simulink model "FixedImpedance"  (R2024b)
settings: Solver=ode4  StartTime=0.001  StopTime=28  FixedStep=1e-4  RelTol=1e-3
libraries: simulink x4, slpidlib x1
settings Model: PacingRate=2  Creator=edwar  LastModifiedBy=edwar

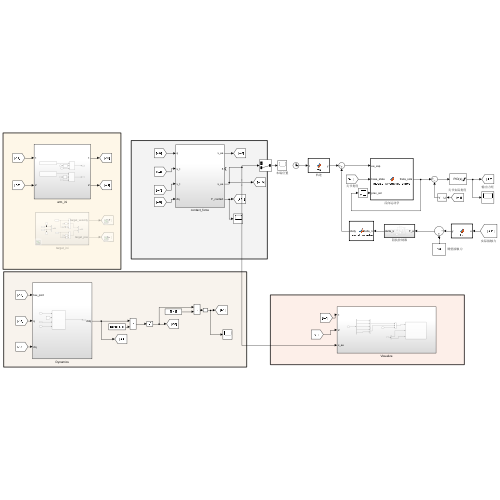
[thumbnail: Simulink's stored preview of the top-level diagram]
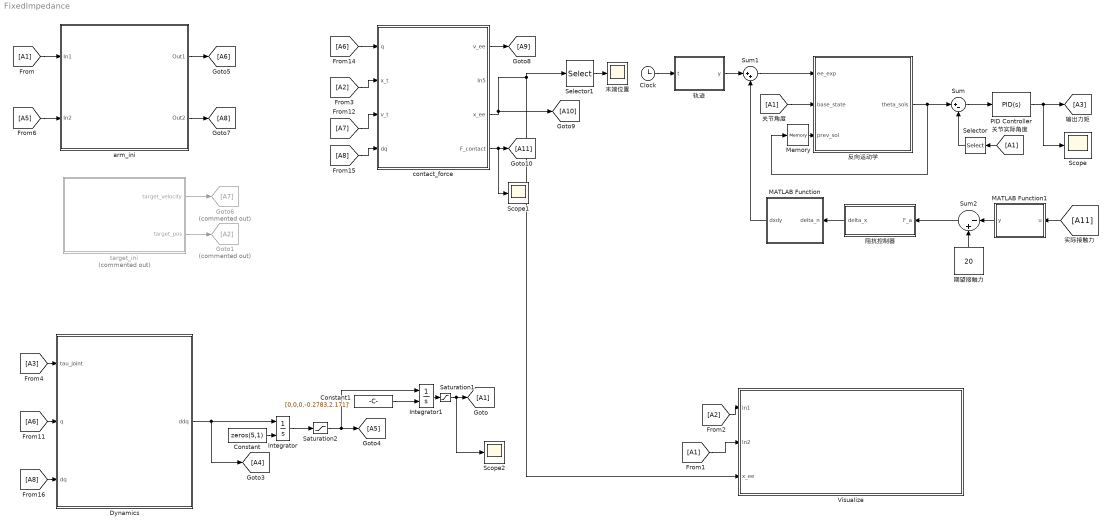
== system FixedImpedance ==
  Clock : Clock
  Constant : Constant  Value=zeros(5,1)
  Constant1 : Constant  Value=[0,0,0,-0.2783,2.171]'
  Dynamics : Subsystem
  Goto1 : Goto  Commented=on  GotoTag=A2
  Goto6 : Goto  Commented=on  GotoTag=A7
  Integrator : Integrator  InitialConditionSource=external  InitialCondition=[0,0,0,0,0]'
  Integrator1 : Integrator  InitialConditionSource=external  InitialCondition=zeros(5,1)
  MATLAB Function : MATLAB Function  TreatAsAtomicUnit=on
  MATLAB Function1 : MATLAB Function  TreatAsAtomicUnit=on
  Memory : Memory  InitialCondition=[0;0]  InheritSampleTime=on
  PID Controller : slpidlib/PID Controller  Controller=PID  Form=Parallel  TimeDomain=Continuous-time  UseExternalTs=off  SampleTime=-1  IntegratorMethod=Forward Euler  FilterMethod=Forward Euler  ControllerParametersSource=internal  P=0.5  I=0  UseKiTs=off  D=0.8  UseExternalDerivativeSource=off  N=100  UseFilter=on  TunerSelectOption=Transfer Function Based (PID Tuner App)  InitialConditionSource=internal  InitialConditionForIntegrator=0  InitialConditionForFilter=0  DifferentiatorICPrevScaledInput=0  ExternalReset=none  TrackingMode=off  Kt=1  LimitOutput=on  SatLimitsSource=internal  UpperSaturationLimit=1.4  LowerSaturationLimit=-1.4  LinearizeAsGain=on  AntiWindupMode=none  Kb=1  LimitIntegrator=off  UpperIntegratorSaturationLimit=inf  LowerIntegratorSaturationLimit=-inf  POutMin=[]  POutMax=[]  IOutMin=[]  IOutMax=[]  DOutMin=[]  DOutMax=[]  NOutMin=[]  NOutMax=[]  SumOutMin=[]  SumOutMax=[]  SaturationOutMin=[]  SaturationOutMax=[]  PParamMin=[]  PParamMax=[]  IParamMin=[]  IParamMax=[]  DParamMin=[]  DParamMax=[]  NParamMin=[]  NParamMax=[]  KbParamMin=[]  KbParamMax=[]  KtParamMin=[]  KtParamMax=[]  KbOutMin=[]  KbOutMax=[]  KtOutMin=[]  KtOutMax=[]  IntegratorOutMin=[]  IntegratorOutMax=[]  FilterOutMin=[]  FilterOutMax=[]  SumI1OutMin=[]  SumI1OutMax=[]  SumI2OutMin=[]  SumI2OutMax=[]  SumI3OutMin=[]  SumI3OutMax=[]  SumI4OutMin=[]  SumI4OutMax=[]  SumDOutMin=[]  SumDOutMax=[]  DifferentiatorOutMin=[]  DifferentiatorOutMax=[]  FilterDiffOutCoefMin=[]  FilterDiffOutCoefMax=[]  ReciprocalOutMin=[]  ReciprocalOutMax=[]  SumDenOutMin=[]  SumDenOutMax=[]  SumNumOutMin=[]  SumNumOutMax=[]  DivideOutMin=[]  DivideOutMax=[]  UdiffTsProdOutMin=[]  UdiffTsProdOutMax=[]  NTsProdOutMin=[]  NTsProdOutMax=[]  UintegralTsProdOutMin=[]  UintegralTsProdOutMax=[]  UngainTsProdOutMin=[]  UngainTsProdOutMax=[]  ClampingZeroOutDataTypeStr=Inherit: Inherit via back propagation  ClampingZeroOutMin=[]  ClampingZeroOutMax=[]  FilterDenConstantOutDataTypeStr=Inherit: Inherit via back propagation  FilterDenConstantOutMin=[]  FilterDenConstantOutMax=[]  PCopyOutDataTypeStr=Inherit: Inherit via back propagation  PCopyOutMin=[]  PCopyOutMax=[]  NCopyOutDataTypeStr=Inherit: Inherit via back propagation  NCopyOutMin=[]  NCopyOutMax=[]  IntegratorContinuousStateAttributes=''  IntegratorStateMustResolveToSignalObject=off  IntegratorRTWStateStorageClass=Auto  FilterContinuousStateAttributes=''  FilterStateMustResolveToSignalObject=off  FilterRTWStateStorageClass=Auto  ParallelPVariant=InternalParameters  IdealPVariant=Disabled  IVariant=InternalParameters  DVariant=InternalParameters  IntegratorVariant=Continuous  SatVariant=Enabled  AWVariant=Passthrough  PCopyVariant=Disabled  TRVariant=Disabled  FdbkBlocksVariant=Forward  IdealPFdbkVariant=Disabled  SatFdbkVariant=Disabled  DerivativeFilterVariant=ContFilter  NVariant=InternalParameters  NCopyVariant=Disabled  FilterICVariant=InternalICsFilter  IntegratorICVariant=InternalICs  ExternalResetVariant=Disabled  TRSumVariant=Passthrough  SumFdbkVariant=Disabled  SumVariant=Sum_PID  TsampFilterVariant=InternalTs  TsampNgainVariant=Passthrough  TsampIntegralVariant=Disabled_SignalSpec  ExternalSaturationOutDataTypeStr=Inherit: Same as second input  DerivativeSourceVariant=ErrorSignal  PreIntVariant=InternalPreInt
  Saturation1 : Saturate  UpperLimit=[1.5,1.5,5*pi,2.5,2.5]'  LowerLimit=[-1.5,-1.5,-5*pi,-2.5,-2.5]'
  Saturation2 : Saturate  UpperLimit=[0.075,0.075,pi/6,4.2,4.2]'  LowerLimit=[-0.075,-0.075,-pi/6,-4.2,-4.2]'
  Scope : Scope
  Scope1 : Scope
  Scope2 : Scope
  Selector : Selector  InputPortWidth=5  IndexOptions=Index vector (dialog)  Indices=[4 5]  OutputSizes=1
  Selector1 : Selector  InputPortWidth=2  IndexOptions=Index vector (dialog)  Indices=[2]  OutputSizes=1
  Sum : Sum  Inputs=|+-
  Sum1 : Sum  Inputs=|++
  Sum2 : Sum  Inputs=|-+
  Visualize : Subsystem
  arm_ini : Subsystem
  contact_force : Subsystem
      settings: PortSchema="{\"entries\":[{\"content\":{\"sides\":[{\"content\":{\"connectorIds\":[\"In1\",\"In2\",\"In3\",\"In4\"]},\"type\":\"ConnectorPlacement.EquallySpacedRectSide\",\"uuid\":\"4288fde3-8199-4324-a6f9-6cd5d2cca29d\"},{\"content\":{\"connectorIds\":[\"Out1\",\"In5\",\"Out2\",\"Out3\"],\"side\":\"RIGHT\"},\"type\":\"ConnectorPlacement.EquallySpacedRectSide\",\"uuid\":\"5c78b4d8-bb77-466a-a925-fe5a2b505b9a\"},{\"content\":{\"side\":\"TOP\"},\"type\":\"ConnectorPlacement.EquallySpacedRectSide\",\"uuid\":\"fef07971-ef14-435e-90c8-30ad3be9ea68\"}]},\"type\":\"ConnectorPlacement.EquallySpacedConnector\",\"uuid\":\"c2bdddc2-d220-4e31-8d95-6807f4723718\"}],\"packageUris\":[\"http://schema.mathworks.com/mf0/Connector/R2020b\"],\"version\":\"1.0\"}"
  target_ini : Subsystem  Commented=on
  反向运动学 : MATLAB Function  TreatAsAtomicUnit=on
  期望接触力 : Constant  Value=20
  末端位置 : Scope
  轨迹 : MATLAB Function  TreatAsAtomicUnit=on
  阻抗控制器 : Subsystem  TreatAsAtomicUnit=on
  wires:
  Saturation2/1 -> Integrator1/1, [A5]
  Saturation1/1 -> Scope2/1, [A1]
  Constant1/1 -> Integrator1/2
  Constant/1 -> Integrator/2
  Integrator1/1 -> Saturation1/1
  Integrator/1 -> Saturation2/1
  Dynamics/1(ddq) -> [A4], Integrator/1
  [A1] -> arm_ini/1(In1)
  [A1] -> Visualize/2(In2)
  [A2] -> Visualize/1(In1)
  [A3] -> Dynamics/1(tau_joint)
  [A5] -> arm_ini/2(In2)
  [A2] -> contact_force/2(x_t)
  target_ini/1(target_velocity) -> Goto6/1
  [A7] -> contact_force/3(v_t)
  target_ini/2(target_pos) -> Goto1/1
  arm_ini/1(Out1) -> [A6]
  [A6] -> Dynamics/2(q)
  [A6] -> contact_force/1(q)
  arm_ini/2(Out2) -> [A8]
  [A8] -> contact_force/4(dq)
  [A8] -> Dynamics/3(dq)
  contact_force/1(v_ee) -> [A9]
  contact_force/2(x_ee) -> Selector1/1, Visualize/3(x_ee), [A10]
  contact_force/3(F_contact) -> Scope1/1, [A11]
  PID Controller/1 -> [A3], Scope/1
  Sum/1 -> PID Controller/1
  [A1] -> Selector/1
  [A1] -> 反向运动学/2(base_state)
  Selector/1 -> Sum/2
  反向运动学/1(theta_sols) -> Memory/1, Sum/1
  阻抗控制器/1(delta_x) -> MATLAB Function/1(delta_n)
  Sum1/1 -> 反向运动学/1(ee_exp)
  [A11] -> MATLAB Function1/1(u)
  期望接触力/1 -> Sum2/2
  Sum2/1 -> 阻抗控制器/1(F_a)
  轨迹/1(y) -> Sum1/1
  Clock/1 -> 轨迹/1(t)
  Memory/1 -> 反向运动学/3(prev_sol)
  MATLAB Function1/1(y) -> Sum2/1
  MATLAB Function/1(dxdy) -> Sum1/2
  Selector1/1 -> 末端位置/1

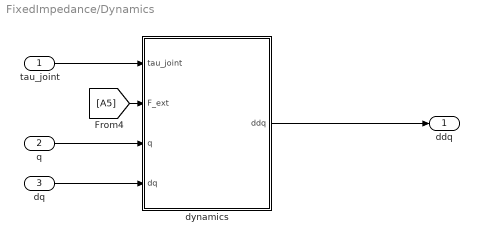
== system FixedImpedance/Dynamics ==
  tau_joint : Inport
  q : Inport  Port=2
  dq : Inport  Port=3
  dynamics : MATLAB Function  TreatAsAtomicUnit=on
  ddq : Outport
  wires:
  tau_joint/1 -> dynamics/1(tau_joint)
  [A5] -> dynamics/2(F_ext)
  dq/1 -> dynamics/4(dq)
  dynamics/1(ddq) -> ddq/1
  q/1 -> dynamics/3(q)

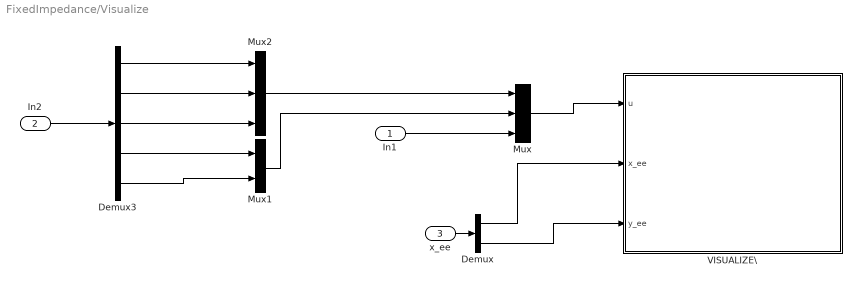
== system FixedImpedance/Visualize ==
  In1 : Inport
  In2 : Inport  Port=2
  x_ee : Inport  Port=3
  Demux : Demux  Outputs=2
  Demux3 : Demux  Outputs=5
  Mux : Mux  Inputs=3
  Mux1 : Mux  Inputs=2
  Mux2 : Mux  Inputs=3
  VISUALIZE\ : MATLAB Function  TreatAsAtomicUnit=on
  wires:
  Demux3/4 -> Mux1/1
  Mux/1 -> VISUALIZE\/1(u)
  Demux3/3 -> Mux2/3
  Mux2/1 -> Mux/1
  Demux3/2 -> Mux2/2
  Mux1/1 -> Mux/2
  Demux3/5 -> Mux1/2
  Demux3/1 -> Mux2/1
  In1/1 -> Mux/3
  In2/1 -> Demux3/1
  x_ee/1 -> Demux/1
  Demux/2 -> VISUALIZE\/3(y_ee)
  Demux/1 -> VISUALIZE\/2(x_ee)

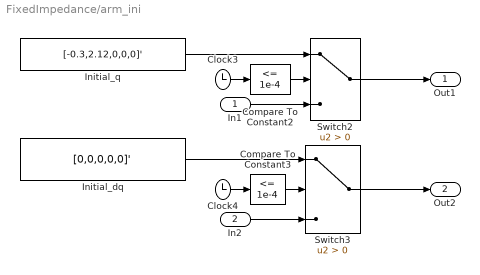
== system FixedImpedance/arm_ini ==
  In1 : Inport
  In2 : Inport  Port=2
  Clock3 : Clock
  Clock4 : Clock
  Compare To Constant2 : simulink/Logic and Bit Operations/Compare To Constant  relop=<=  const=1e-4  OutDataTypeStr=boolean
  Compare To Constant3 : simulink/Logic and Bit Operations/Compare To Constant  relop=<=  const=1e-4  OutDataTypeStr=boolean
  Initial_dq : Constant  Value=[0,0,0,0,0]'
  Initial_q : Constant  Value=[-0.3,2.12,0,0,0]'
  Switch2 : Switch  Criteria=u2 > Threshold  SaturateOnIntegerOverflow=off  InputSameDT=off
  Switch3 : Switch  Criteria=u2 > Threshold  SaturateOnIntegerOverflow=off  InputSameDT=off
  Out1 : Outport
  Out2 : Outport  Port=2
  wires:
  In1/1 -> Switch2/3
  Compare To Constant3/1 -> Switch3/2
  Switch3/1 -> Out2/1
  Initial_dq/1 -> Switch3/1
  Clock3/1 -> Compare To Constant2/1
  In2/1 -> Switch3/3
  Clock4/1 -> Compare To Constant3/1
  Initial_q/1 -> Switch2/1
  Compare To Constant2/1 -> Switch2/2
  Switch2/1 -> Out1/1

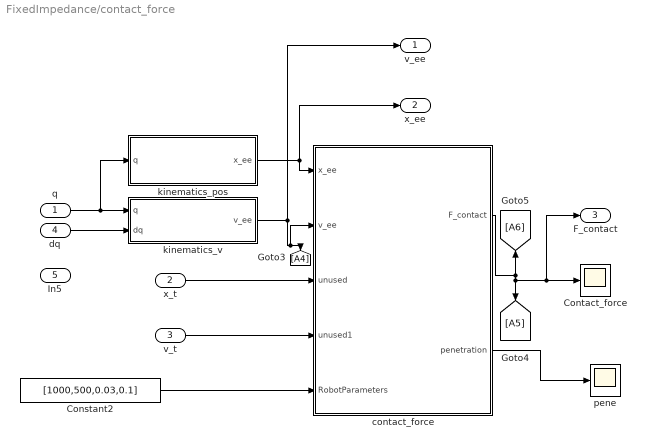
== system FixedImpedance/contact_force ==
  q : Inport
  x_t : Inport  Port=2
  v_t : Inport  Port=3
  dq : Inport  Port=4
  In5 : Inport  Port=5
  Constant2 : Constant  Value=[1000,500,0.03,0.1]
  Contact_force : Scope
  contact_force : MATLAB Function  TreatAsAtomicUnit=on  SystemSampleTime=0.01
  kinematics_pos : MATLAB Function  TreatAsAtomicUnit=on
  kinematics_v : MATLAB Function  TreatAsAtomicUnit=on
  pene : Scope
  v_ee : Outport
  x_ee : Outport  Port=2
  F_contact : Outport  Port=3
  wires:
  kinematics_v/1(v_ee) -> v_ee/1, contact_force/2(v_ee), [A4]
  contact_force/1(F_contact) -> [A5], Contact_force/1, F_contact/1, [A6]
  kinematics_pos/1(x_ee) -> x_ee/1, contact_force/1(x_ee)
  x_t/1 -> contact_force/3(unused)
  Constant2/1 -> contact_force/5(RobotParameters)
  q/1 -> kinematics_pos/1(q), kinematics_v/1(q)
  v_t/1 -> contact_force/4(unused1)
  dq/1 -> kinematics_v/2(dq)
  contact_force/2(penetration) -> pene/1

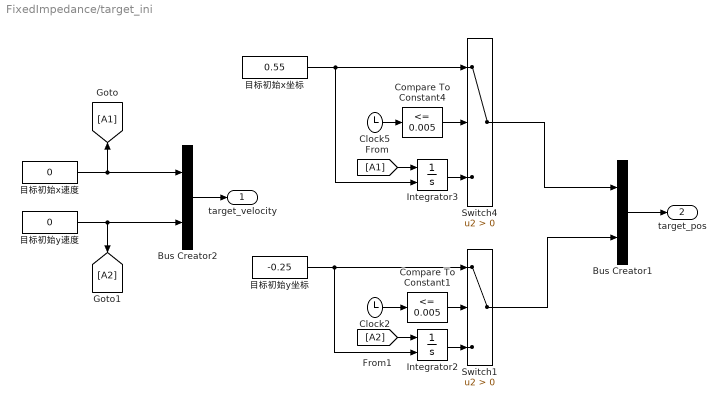
== system FixedImpedance/target_ini ==
  Bus Creator1 : BusCreator  Inputs=2
  Bus Creator2 : BusCreator  Inputs=2
  Clock2 : Clock
  Clock5 : Clock
  Compare To Constant1 : simulink/Logic and Bit Operations/Compare To Constant  relop=<=  const=0.005  OutDataTypeStr=boolean
  Compare To Constant4 : simulink/Logic and Bit Operations/Compare To Constant  relop=<=  const=0.005  OutDataTypeStr=boolean
  Integrator2 : Integrator  InitialConditionSource=external
  Integrator3 : Integrator  InitialConditionSource=external
  Switch1 : Switch  Criteria=u2 > Threshold  SaturateOnIntegerOverflow=off  InputSameDT=off
  Switch4 : Switch  Criteria=u2 > Threshold  SaturateOnIntegerOverflow=off  InputSameDT=off
  目标初始x坐标 : Constant  Value=0.55
  目标初始x速度 : Constant  Value=0
  目标初始y坐标 : Constant  Value=-0.25
  目标初始y速度 : Constant  Value=0
  target_velocity : Outport
  target_pos : Outport  Port=2
  wires:
  Compare To Constant4/1 -> Switch4/2
  Integrator2/1 -> Switch1/3
  Integrator3/1 -> Switch4/3
  目标初始x速度/1 -> [A1], Bus Creator2/1
  目标初始x坐标/1 -> Switch4/1, Integrator3/2
  目标初始y坐标/1 -> Switch1/1, Integrator2/2
  目标初始y速度/1 -> [A2], Bus Creator2/2
  Compare To Constant1/1 -> Switch1/2
  Switch4/1 -> Bus Creator1/1
  Clock5/1 -> Compare To Constant4/1
  Clock2/1 -> Compare To Constant1/1
  Switch1/1 -> Bus Creator1/2
  Bus Creator2/1 -> target_velocity/1
  Bus Creator1/1 -> target_pos/1
  [A1] -> Integrator3/1
  [A2] -> Integrator2/1

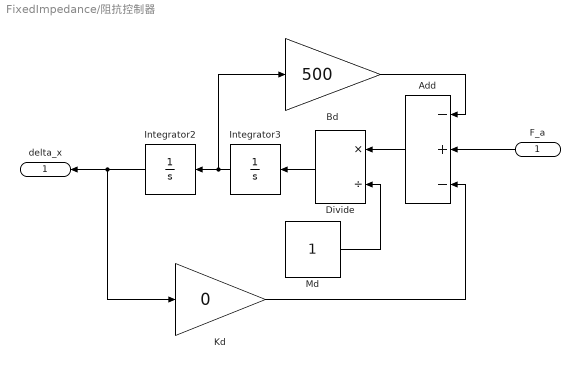
== system FixedImpedance/阻抗控制器 ==
  F_a : Inport
  Add : Sum  Inputs=-+-
  Bd : Gain  Gain=500
  Divide : Product  Inputs=*/
  Integrator2 : Integrator
  Integrator3 : Integrator
  Kd : Gain  Gain=0
  Md : Constant
  delta_x : Outport
  wires:
  Md/1 -> Divide/2
  Bd/1 -> Add/1
  Integrator3/1 -> Integrator2/1, Bd/1
  Kd/1 -> Add/3
  Add/1 -> Divide/1
  F_a/1 -> Add/2
  Integrator2/1 -> delta_x/1, Kd/1
  Divide/1 -> Integrator3/1

== matlab function FixedImpedance/Dynamics/dynamics ==
  data: tau_joint input; F_ext input size=[2,1]; q input size=[5,1]; ddq output size=[5,1]; dq input size=[5,1]
function ddq  = robot_dynamics(tau_joint, F_ext, q, dq)
    % 平面二连杆机器人动力学模型
    % 输入: tau_joint (2x1), F_ext (2x1?), q (5x1), dq (5x1?)
    % 输出: ddq (5x1)


    % 构建力矩向量（5维，前三个分量为0，假设前3是基座自由度不受控）
    tau_control = zeros(5,1);
    tau_control(4:5) = tau_joint(:);  % 关节控制力矩

    J = jacobian_matrix(q);

    % 接触力映射到关节空间
    if ~isempty(F_ext)
        tau_contact = -J' * F_ext(:);
    else
        tau_contact = zeros(5,1);
    end

    tau_total = tau_control + tau_contact;
    damping_coeff = 0.05;  % 0.02 ~ 0.1
    tau_damping = -damping_coeff * dq;  % 5x1，对所有自由度加线性阻尼
    tau_total = tau_total + tau_damping;
    [D, C] = dynamics_model(q, dq); 
    det_D = det(D);
    cond_D = cond(D);
    % 加速度
    ddq = D \ (tau_total - C);
end

== matlab function FixedImpedance/contact_force/kinematics_pos ==
  data: x_ee output; q input
function x_ee  = forward_kinematics(q)
    x_ee = zeros(1,2);
    % q = [x_b; y_b; theta_b; theta1; theta2]
    x_b = q(1); y_b = q(2); theta_b = q(3);
    theta1 = q(4); theta2 = q(5);
    b_b = 0.151;
    L1 = 0.225; L2 = 0.276;  % 连杆长度
    
    % 相对基座的末端位置
    x_rel = b_b + L1*cos(theta1) + L2*cos(theta1+theta2);
    y_rel = L1*sin(theta1) + L2*sin(theta1+theta2);
    
    % 转换到世界坐标系
    R = [cos(theta_b) -sin(theta_b); sin(theta_b) cos(theta_b)];
    pos_world = R * [x_rel; y_rel] + [x_b; y_b];
    
    x_ee(1) = pos_world(1);
    x_ee(2) = pos_world(2);
end

== matlab function FixedImpedance/contact_force/contact_force ==
  data: x_ee input; F_contact output double size=[2,1]; v_ee input; unused input; unused1 input; RobotParameters input; penetration output
function [F_contact,penetration] = contact_force(x_ee, v_ee, ~, ~, RobotParameters)
    % 预分配接触力
    F_contact = zeros(2,1);   
    x_ee = x_ee(:);
    v_ee = v_ee(:);
    
    % 提取参数
    K    = RobotParameters(1);
    B    = RobotParameters(2);
    R_ee = RobotParameters(3); % 末端工具半径
    
    %% 正弦曲面参数 (固定墙体在上方，高度带有 0.2 偏移)

    y = x_ee(2);
    
    %% 1. 计算当前 X 位置对应的曲面 Y 高度
    % 纯 Y 方向模型不需要计算导数 dydx 了
    y_surface = 0.2;
    
    %% 2. 计算纯 Y 方向的穿透深度
    % 机械臂在下方，最上沿的坐标是 y + R_ee
    % 当最上沿超过曲面高度时，发生接触
    penetration = (y + R_ee) - y_surface;
    
    if penetration > 0
        %% 3. 计算沿 Y 方向挤压墙体的速度
        % v_ee(2) 是末端在世界坐标系 Y 方向的速度
        % 因为墙在上方，向上运动（vy > 0）代表正在挤入墙体
        v_in = v_ee(2); 
        
        %% 4. 计算接触力的大小
        F_spring = K * penetration;
        F_damp   = B * max(v_in, 0); % 只有向上挤压墙体时才产生阻尼力
        
        %% 5. 输出接触力向量（方向绝对沿世界坐标 Y 轴向下）
        % 墙体在上方，给机械臂的弹力与阻尼力必然是垂直向下的
        F_contact(1) = 0;                  % X 方向不受力
        F_contact(2) = -(F_spring + F_damp); % Y 方向受力向下
    end
end

== matlab function FixedImpedance/contact_force/kinematics_v ==
  data: q input; v_ee output; dq input
function v_ee = forward_kinematics_v(q,dq)
J = jacobian_matrix(q);
% 计算末端速度
v_ee = (J * dq)';
end

== matlab function FixedImpedance/Visualize/VISUALIZE\ ==
  settings: updateMethod=DISCRETE
  data: u input; x_ee input; y_ee input
function visualize_arm(u,x_ee,y_ee)

% ================================================
% 平面二连杆自由基座机械臂 + 水平墙面 可视化（Simulink专用）
% 输入 u = [x_b, y_b, theta_b, q1, q2, x_ee, y_ee]
%       前5个：用于绘制机械臂本体
%       后2个：直接传入的末端执行器位置，用于绘制轨迹
% ================================================

% ================== 参数（直接使用您提供的值） ==================
b_b   = 0.151;   % 基座质心到关节1距离 (m)
l1    = 0.225;   % 连杆1长度 (m)
l2    = 0.276;   % 连杆2长度 (m)
R_ee  = 0.03;    % 末端执行器半径 (m)

% ================== 持久化图形对象（只创建一次） ==================
persistent h_fig h_base h_link1 h_link2 h_ee h_surface ...
           ee_offset_x ee_offset_y base_vertices
persistent call_counter visualize_every
persistent h_traj traj_x traj_y max_traj_points traj_idx  % 轨迹相关

if isempty(call_counter)
    call_counter = 0;
    visualize_every = 50;
end

call_counter = call_counter + 1;
if mod(call_counter, visualize_every) ~= 0
    return;
end

if isempty(h_fig)
    h_fig = figure();
    ax = gca;
    hold(ax, 'on');
    grid(ax, 'on');
    axis(ax, 'equal');
    xlim(ax, [-0.5 1]);
    ylim(ax, [-0.5 1]);
    xlabel(ax, 'X (m)');
    ylabel(ax, 'Y (m)');
    
    % 初始化基座线段
    base_size = 0.28;           
    half = base_size / 2;
    base_vertices = [ ...
        -half, -half;
         half, -half;
         half,  half;
        -half,  half;
        -half, -half];
    
    % 创建基座
    h_base = patch(ax, ...
        'XData', base_vertices(:,1), 'YData', base_vertices(:,2), ...
        'FaceColor', 'k', ...     
        'EdgeColor', [0.5 0.5 0.5], ...            
        'LineWidth', 2.5, ...
        'FaceAlpha', 0.85);
        
    h_link1 = line(ax, [0 0], [0 0], 'Color', [0.5 0.5 0.5], 'LineWidth', 4, 'DisplayName', 'L1');
    h_link2 = line(ax, [0 0], [0 0], 'Color', [0.5 0.5 0.5], 'LineWidth', 4, 'DisplayName', 'L2');
    
    % 末端执行器圆圈
    theta_c = linspace(0, 2*pi, 50);
    ee_offset_x = R_ee * cos(theta_c);
    ee_offset_y = R_ee * sin(theta_c);
    h_ee = line(ax, ee_offset_x, ee_offset_y, ...
                'Color', 'b', 'LineWidth', 1.5);
                     
    x_surface = linspace(-0.5, 1, 500);
    y_surface = 0.2;
    h_surface = line(ax, x_surface, y_surface, ...
                     'Color', 'k', ...         % 'r' 改为 'k' (黑色)
                     'LineStyle', '--', ...    % 新增：设置为虚线
                     'LineWidth', 1.5);
    
    % 【新增】初始化轨迹线
    h_traj = line(ax, nan, nan, ...
                  'Color', [0 0 1], ...      % 深绿色
                  'LineWidth', 1.5, ...
                  'LineStyle', '--');
    
    % 【新增】初始化轨迹存储
    max_traj_points = 10000;
    traj_x = nan(max_traj_points, 1);
    traj_y = nan(max_traj_points, 1);
    traj_idx = 1;
    
end

% ================== 提取输入 ==================
xb     = u(1);
yb     = u(2);
thetab = u(3);
q1     = u(4);
q2     = u(5);


% ================== 正运动学（用于绘制连杆，不含末端） ==================
x_j1 = xb + b_b * cos(thetab);
y_j1 = yb + b_b * sin(thetab);
x_j2 = x_j1 + l1 * cos(thetab + q1);
y_j2 = y_j1 + l1 * sin(thetab + q1);
% 注意：这里不再计算 x_ee, y_ee，而是直接使用传入的

% ================== 更新轨迹（使用传入的末端位置） ==================
traj_x(traj_idx) = x_ee;
traj_y(traj_idx) = y_ee;

traj_idx = traj_idx + 1;
if traj_idx > max_traj_points
    traj_idx = 1;
end

% 获取有效轨迹数据
if traj_idx > 1
    valid_x = traj_x(1:traj_idx-1);
    valid_y = traj_y(1:traj_idx-1);
else
    valid_x = traj_x;
    valid_y = traj_y;
end
set(h_traj, 'XData', valid_x, 'YData', valid_y);

% ================== 更新图形 ==================
R = [cos(thetab), -sin(thetab); 
     sin(thetab),  cos(thetab)];
 
rotated = (R * base_vertices')';          
abs_x = xb + rotated(:,1);
abs_y = yb + rotated(:,2);

set(h_base, 'XData', abs_x, 'YData', abs_y);
set(h_link1, 'XData', [x_j1, x_j2], 'YData', [y_j1, y_j2]);
set(h_link2, 'XData', [x_j2, x_ee], 'YData', [y_j2, y_ee]);  % 使用传入的末端位置
set(h_ee,    'XData', x_ee + ee_offset_x, 'YData', y_ee + ee_offset_y);  % 使用传入的末端位置

drawnow limitrate;

end

== matlab function FixedImpedance/反向运动学 ==
  data: ee_exp input; theta_sols output; base_state input; prev_sol input
function theta_sols = inverse_kinematics_stable(ee_exp, base_state, prev_sol)
    %#codegen
    b_b = 0.151; L1 = 0.225; L2 = 0.276;
    
    x_t = ee_exp(1); y_t = ee_exp(2);
    x_b = base_state(1); y_b = base_state(2); theta_b = base_state(3);
    
    % 当前关节角（带保护）
    if length(base_state) >= 5
        q_current = [base_state(4); base_state(5)];
    else
        q_current = [0; 0];
    end
    
    % 使用上一次成功解作为参考，确保是列向量
    if nargin < 3 || isempty(prev_sol)
        ref = q_current(:);  % 确保是列向量
    else
        ref = prev_sol(:);   % 确保是列向量
    end
   
    
    % 坐标变换
    dx = x_t - x_b; dy = y_t - y_b;
    x_prime = cos(theta_b)*dx + sin(theta_b)*dy - b_b;
    y_prime = -sin(theta_b)*dx + cos(theta_b)*dy;
    
    r_sq = x_prime^2 + y_prime^2;
    r = sqrt(r_sq);
    
    % 可达性检查
    if r > (L1 + L2) || r < abs(L1 - L2) || r < 1e-6
        theta_sols = ref(:);  % 确保输出是列向量
        return;
    end
    
    cos_theta2 = (r_sq - L1^2 - L2^2) / (2 * L1 * L2);
    cos_theta2 = max(-1.0, min(1.0, cos_theta2));
    
    sin_theta2 = sqrt(1 - cos_theta2^2);   % 正值
    
    angle_base = atan2(y_prime, x_prime);
    
    % 两组解（确保都是列向量）
    theta2_a = atan2( sin_theta2, cos_theta2);
    theta2_b = atan2(-sin_theta2, cos_theta2);
    
    theta1_a = angle_base - atan2(L2*sin_theta2, L1 + L2*cos_theta2);
    theta1_b = angle_base - atan2(-L2*sin_theta2, L1 + L2*cos_theta2);
    
    sol_a = [theta1_a; theta2_a];
    sol_b = [theta1_b; theta2_b];
    
    % ================== 关键改进：连续性处理 ==================
    % 1. 先把两组解都缠绕到最接近参考解
    sol_a = ref + wrapToPi(sol_a - ref);
    sol_b = ref + wrapToPi(sol_b - ref);
    
    % 2. 计算代价（距离 + 配置切换惩罚）
    % 现在ref(1)和ref(2)都可以安全访问
    cost_a = sum((sol_a - ref).^2) + 0.5 * abs(sol_a(2) - ref(2));
    cost_b = sum((sol_b - ref).^2) + 0.5 * abs(sol_b(2) - ref(2));  
    % 3. 优先选择最接近的
    if cost_a <= cost_b
        theta_sols = sol_a;
    else
        theta_sols = sol_b;
    end
    
    % 最终再对当前状态做一次小调整（防止累计漂移）
    theta_sols = ref + wrapToPi(theta_sols - ref);
    theta_sols = theta_sols(:);  % 确保输出是列向量
end

== matlab function FixedImpedance/MATLAB Function ==
  data: delta_n input; dxdy output
function dxdy = sinusoidal_impedance(delta_n)
    dxdy = zeros(2, 1);
%#codegen

    % X 方向不作任何阻抗修正，防止前进方向死锁
    dxdy(1) = 0; 
    
    % Y 方向直接赋修正量
    % 注：如果你的 delta_n 物理意义是指向“上方”为正，而你想让它往下压，这里可以加负号（-delta_n）
    dxdy(2) = delta_n; 
    
end
% % 正弦曲线接触面的阻抗修正
%     %
%     % 输入:
%     %   delta_n - 法向修正量（标量）
%     %   x_t, y_t - 实际末端位置（世界坐标）
%     %   x_b, y_b, theta_b - 基座状态
%     %   b_b - 基座偏移
%     %   A - 正弦曲线幅值
%     %   omega - 正弦曲线频率
%     %   phi - 正弦曲线相位
%     %
%     % 输出:
%     %   dx, dy - XY方向修正量（世界坐标）
% 
% 
% function dxdy = sinusoidal_impedance(delta_n, ee_target,base_state)
%     dxdy=zeros(2,1);
% %#codegen
%     % 简化版：直接计算当前x位置的法向量
%     x_b = base_state(1);
%     y_b = base_state(2);
%     theta_b = base_state(3);
%     b_b = 0.151;
%     omega = 2*pi/0.3;
%     A = 0.05;
%     phi = 0;
%     x_t = ee_target(1);
%     y_t = ee_target(2);
%     % 转换到基座坐标系
%     dx_world = x_t - x_b;
%     dy_world = y_t - y_b;
% 
%     x_body = cos(theta_b)*dx_world + sin(theta_b)*dy_world - b_b;
% 
%     % 导数
%     dy_dx_surface = A * omega * cos(omega * x_body + phi);
% 
%     % % 法向量（指向远离曲线的方向）
%     nx_body = dy_dx_surface;
%     ny_body = -1;
%     % 归一化
%     norm_val = sqrt(nx_body^2 + ny_body^2);
%     nx_body = nx_body / norm_val;
%     ny_body = ny_body / norm_val;
% 
%     % 转换到世界坐标
%     nx_world = cos(theta_b)*nx_body - sin(theta_b)*ny_body;
%     ny_world = sin(theta_b)*nx_body + cos(theta_b)*ny_body;
% 
%     % 计算修正量
%     dxdy(1) = delta_n * nx_world;
%     dxdy(2) = delta_n * ny_world;
% end

== matlab function FixedImpedance/MATLAB Function1 ==
  data: u input; y output
function y = fcn(u)
    y = abs(u(2));
end

== matlab function FixedImpedance/轨迹 ==
  data: t input; y output
function y = fcn(t)
    v = 0.01;   % x方向运动速度
    x_start = 0.28;
    x_stop  = 0.58;

    % 计算不受限制的 x 位置
    x = x_start + v * t;
    
    % 限制在 0.65
    if x > x_stop
        x = x_stop;
    end
    
    y = zeros(2,1);
    y(1) = x;
    y(2) = 0.2;
end
